simulink model "Mpc_test"  (R2018b)
settings: Solver=VariableStepAuto  StartTime=0.0  StopTime=40  RelTol=1e-3
libraries: mpclib x1
settings Model: Creator=erange  LastModifiedBy=erange

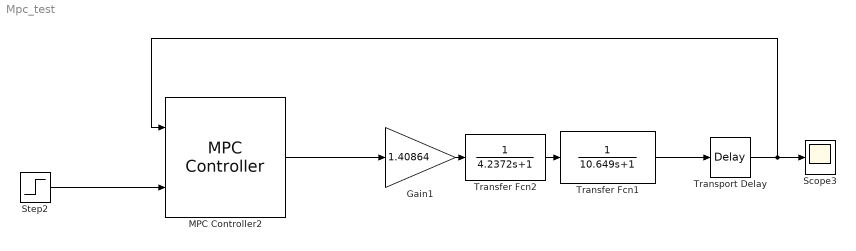
== system Mpc_test ==
  Gain1 : Gain  Gain=1.40864
  MPC Controller2 : mpclib/MPC Controller  SCDEnableBlockLinearizationSpecification=on  mpcobj=mpc2  is_multiple=0  enable_value=0  return_u0=off  updateMPCinCallerWorkspace=on  md_inport=off  mv_inport=off  return_cost=off  return_mvseq=off  return_qpstatus=off  return_xseq=off  return_state=off  return_ovseq=off  state_inport=off  umin_inport=off  umax_inport=off  ymin_inport=off  ymax_inport=off  cc_inport=off  ywt_inport=off  uwt_inport=off  duwt_inport=off  rhoeps_inport=off  uref_inport=off  n_ts=0.01  n_p=500  n_mv=1  n_md=0  n_ud=0  n_mo=1  n_uo=0  BlockDataType=double  SampleTimeInherited=off  switch_inport=off
  Scope3 : Scope
  Step2 : Step  Time=0  SampleTime=1
  Transfer Fcn1 : TransferFcn  Denominator=[10.649 1]
  Transfer Fcn2 : TransferFcn  Denominator=[4.2372 1]
  Transport Delay : TransportDelay  DelayTime=3
  wires:
  MPC Controller2/1 -> Gain1/1
  Step2/1 -> MPC Controller2/2
  Transfer Fcn2/1 -> Transfer Fcn1/1
  Gain1/1 -> Transfer Fcn2/1
  Transfer Fcn1/1 -> Transport Delay/1
  Transport Delay/1 -> MPC Controller2/1, Scope3/1
